simulink model "leader_follower"  (R2017b)
settings: Solver=FixedStepDiscrete  StartTime=0.0  StopTime=inf  FixedStep=0.1  RelTol=1e-3  EnableMultiTasking=on
undefined symbols (not defined in the file): Angular, Linear
libraries: robotlib x4, realtime_pacer_lib x1
settings Model: Creator=The MathWorks, Inc.  LastModifiedBy=bsb
settings DataIOCC: LimitDataPoints=on  SaveFormat=Array
settings OptimizationCC: DefaultUnderspecifiedDataType=single  LifeSpan=1  MaxStackSize=64
settings DebuggingCC: SolverPrmCheckMsg=warning  SFUnexpectedBacktrackingDiag=warning  SFNoUnconditionalDefaultTransitionDiag=warning  SFExecutionAtInitializationDiag=none
settings HardwareCC: ProdBitPerPointer=32  ProdBitPerSizeT=32  ProdBitPerPtrDiffT=32  ProdLargestAtomicFloat=None  ProdIntDivRoundTo=Undefined  ProdEndianess=Unspecified  ProdWordSize=32  ProdHWDeviceType=Generic->Unspecified (assume 32-bit Generic)  TargetHWDeviceType=Generic->Unspecified (assume 32-bit Generic)  UseEmbeddedCoderFeatures=off
settings ModelReferenceCC: PropagateSignalLabelsOutOfModel=off
settings RTWCC: SystemTargetFile=ert.tlc  HardwareBoard=Robot Operating System (ROS)  TLCOptions=-aInlineSetEventsForThisBaseRateFcn=TLC_FALSE -aSuppressMultiTaskScheduler=TLC_FALSE -aRateBasedStepFcn=0  TemplateMakefile=ert_default_tmf  Toolchain=Catkin  TargetLang=C++
settings CodeAppCC: StateflowObjectComments=on
settings ERTTargetCC: MultiwordLength=2048  ERTCustomFileBanners=off  MultiInstanceERTCode=on  CodeInterfacePackaging=C++ class  SupportContinuousTime=on  SupportNonInlinedSFcns=on  RemoveResetFunc=off  SupportVariableSizeSignals=on  ModelStepFunctionPrototypeControlCompliant=off  RootIOFormat=Structure reference  ConvertIfToSwitch=off  SuppressUnreachableDefaultCases=off
settings ConfigComp: CovMetricSettings=dw  CovHtmlReporting=on  CovSaveCumulativeToWorkspaceVar=on  CovSaveSingleToWorkspaceVar=on  CovExternalEMLEnable=off  CovSFcnEnable=off

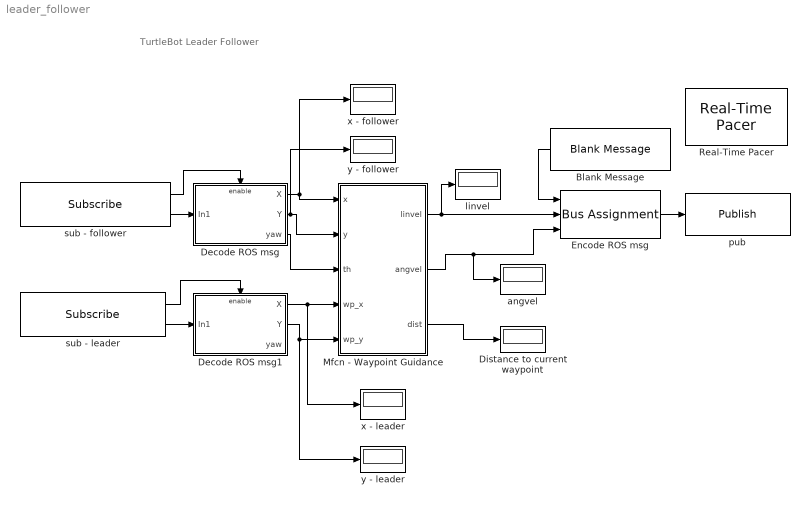
== system leader_follower ==
  note: TurtleBot Leader Follower
  Blank Message : robotlib/Blank Message  SourceLibraryInfo=This block requires Robotics System Toolbox  messageType=geometry_msgs/Twist  SampleTime=inf
      settings: SourceProductBaseCode=RO
  Decode ROS msg : Subsystem
  Decode ROS msg1 : Subsystem
  Distance to current waypoint : Display
  Encode ROS msg : BusAssignment  AssignedSignals=Linear.X,Angular.Z
  Mfcn - Waypoint Guidance : MATLAB Function  TreatAsAtomicUnit=on
  Real-Time Pacer : realtime_pacer_lib/Real-Time Pacer  simTimePerRealTime=1
  angvel : Display
  linvel : Display
  pub : robotlib/Publish  SourceLibraryInfo=This block requires Robotics System Toolbox  topicSource=Select from ROS network  topic=/tb3_1/cmd_vel  messageType=geometry_msgs/Twist  messageQueueLength=105
      settings: SourceProductBaseCode=RO
  "sub - follower " : robotlib/Subscribe  SourceLibraryInfo=This block requires Robotics System Toolbox  topicSource=Select from ROS network  topic=/tb3_1/amcl_pose  messageType=geometry_msgs/PoseWithCovarianceStamped  sampleTime=-1  messageQueueLength=51
      settings: SourceProductBaseCode=RO
  sub - leader : robotlib/Subscribe  SourceLibraryInfo=This block requires Robotics System Toolbox  topicSource=Select from ROS network  topic=/tb3_0/amcl_pose  messageType=geometry_msgs/PoseWithCovarianceStamped  sampleTime=-1  messageQueueLength=51
      settings: SourceProductBaseCode=RO
  x - follower : Display
  x - leader : Display
  y - follower : Display
  y - leader : Display
  wires:
  Encode ROS msg/1 -> pub/1
  "sub - follower "/1 -> Decode ROS msg/Enable
  "sub - follower "/2 -> Decode ROS msg/1(In1)
  Blank Message/1 -> Encode ROS msg/1
  Decode ROS msg/1(X) -> Mfcn - Waypoint Guidance/1(x), x - follower/1
  Decode ROS msg/2(Y) -> y - follower/1, Mfcn - Waypoint Guidance/2(y)
  Mfcn - Waypoint Guidance/3(dist) -> Distance to current waypoint/1
  Decode ROS msg1/1(X) -> x - leader/1, Mfcn - Waypoint Guidance/4(wp_x)
  Decode ROS msg/3(yaw) -> Mfcn - Waypoint Guidance/3(th)
  Mfcn - Waypoint Guidance/2(angvel) -> angvel/1, Encode ROS msg/3
  Mfcn - Waypoint Guidance/1(linvel) -> linvel/1, Encode ROS msg/2
  sub - leader/2 -> Decode ROS msg1/1(In1)
  Decode ROS msg1/2(Y) -> y - leader/1, Mfcn - Waypoint Guidance/5(wp_y)
  sub - leader/1 -> Decode ROS msg1/Enable

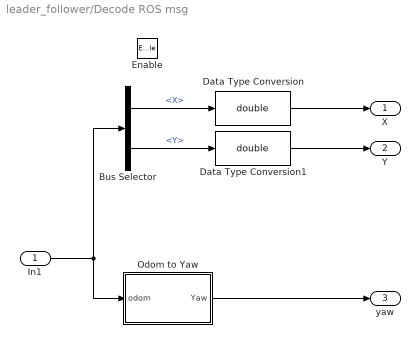
== system leader_follower/Decode ROS msg ==
  In1 : Inport
  Enable : EnablePort
  Bus Selector : BusSelector  DialogController=Simulink.DDGSource_BusSelector  OutputSignals=Pose.Pose.Position.X,Pose.Pose.Position.Y
  Data Type Conversion : DataTypeConversion  OutDataTypeStr=double
  Data Type Conversion1 : DataTypeConversion  OutDataTypeStr=double
  Odom to Yaw : Subsystem
  X : Outport
  Y : Outport  Port=2
  yaw : Outport  Port=3
  wires:
  In1/1 -> Odom to Yaw/1(odom), Bus Selector/1
  Bus Selector/2 -> Data Type Conversion1/1  "<Y>"
  Bus Selector/1 -> Data Type Conversion/1  "<X>"
  Data Type Conversion/1 -> X/1
  Data Type Conversion1/1 -> Y/1
  Odom to Yaw/1(Yaw) -> yaw/1

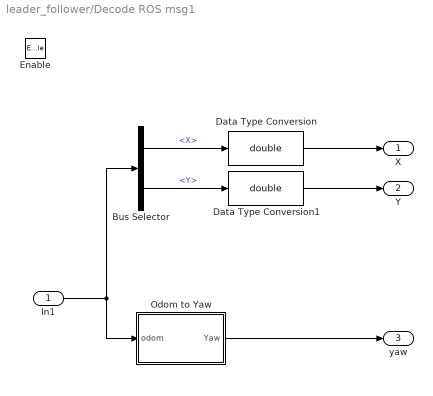
== system leader_follower/Decode ROS msg1 ==
  In1 : Inport
  Enable : EnablePort
  Bus Selector : BusSelector  DialogController=Simulink.DDGSource_BusSelector  OutputSignals=Pose.Pose.Position.X,Pose.Pose.Position.Y
  Data Type Conversion : DataTypeConversion  OutDataTypeStr=double
  Data Type Conversion1 : DataTypeConversion  OutDataTypeStr=double
  Odom to Yaw : Subsystem
  X : Outport
  Y : Outport  Port=2
  yaw : Outport  Port=3
  wires:
  In1/1 -> Odom to Yaw/1(odom), Bus Selector/1
  Bus Selector/2 -> Data Type Conversion1/1  "<Y>"
  Bus Selector/1 -> Data Type Conversion/1  "<X>"
  Data Type Conversion/1 -> X/1
  Data Type Conversion1/1 -> Y/1
  Odom to Yaw/1(Yaw) -> yaw/1

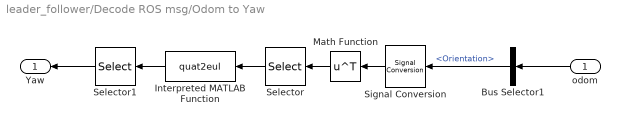
== system leader_follower/Decode ROS msg/Odom to Yaw ==
  odom : Inport
  Bus Selector1 : BusSelector  OutputSignals=Pose.Pose.Orientation
  Interpreted MATLAB Function : MATLABFcn  MATLABFcn=quat2eul  OutputDimensions=3
  Math Function : Math  Operator=transpose  SaturateOnIntegerOverflow=on
  Selector : Selector  InputPortWidth=4  IndexOptions=Index vector (dialog)  Indices=[4 1 2 3]  OutputSizes=1
  Selector1 : Selector  InputPortWidth=3  IndexOptions=Index vector (dialog)  Indices=1  OutputSizes=1
  Signal Conversion : SignalConversion  ConversionOutput=Virtual bus  OverrideOpt=off
  Yaw : Outport
  wires:
  odom/1 -> Bus Selector1/1
  Bus Selector1/1 -> Signal Conversion/1  "<Orientation>"
  Selector/1 -> Interpreted MATLAB Function/1
  Interpreted MATLAB Function/1 -> Selector1/1
  Selector1/1 -> Yaw/1
  Math Function/1 -> Selector/1
  Signal Conversion/1 -> Math Function/1

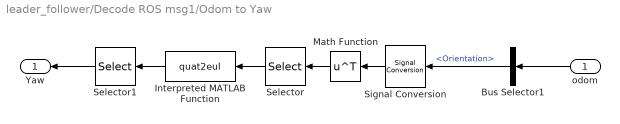
== system leader_follower/Decode ROS msg1/Odom to Yaw ==
  odom : Inport
  Bus Selector1 : BusSelector  OutputSignals=Pose.Pose.Orientation
  Interpreted MATLAB Function : MATLABFcn  MATLABFcn=quat2eul  OutputDimensions=3
  Math Function : Math  Operator=transpose  SaturateOnIntegerOverflow=on
  Selector : Selector  InputPortWidth=4  IndexOptions=Index vector (dialog)  Indices=[4 1 2 3]  OutputSizes=1
  Selector1 : Selector  InputPortWidth=3  IndexOptions=Index vector (dialog)  Indices=1  OutputSizes=1
  Signal Conversion : SignalConversion  ConversionOutput=Virtual bus  OverrideOpt=off
  Yaw : Outport
  wires:
  odom/1 -> Bus Selector1/1
  Bus Selector1/1 -> Signal Conversion/1  "<Orientation>"
  Selector/1 -> Interpreted MATLAB Function/1
  Interpreted MATLAB Function/1 -> Selector1/1
  Selector1/1 -> Yaw/1
  Math Function/1 -> Selector/1
  Signal Conversion/1 -> Math Function/1

== matlab function leader_follower/Mfcn - Waypoint Guidance ==
  data: linvel output; angvel output; x input; dist output; y input; th input; wp_x input; wp_y input
function [linvel,angvel,dist] = wpt_fcn(x,y,th,wp_x,wp_y)
% Function to implement waypoint guidance
% Inputs:
%  - x: Current X position
%  - y: Current Y position
%  - th: Current theta position
%  - wp_x: Current waypoint goals, X
%  - wp_y: Current waypoint goals, X
% Outputs:
%  - dist: Distance from current position to current waypoint goal
%  - angvel: Desired angular velocity [rad/s, clockwise]
%  - linvel: Desired linear velocity


% Distance from waypoint to current location
dist = sqrt((x-wp_x)^2+(y-wp_y)^2);

% Angle from current location to waypoint
course = atan2(wp_y-y,wp_x-x);

% Difference (error) between current turtle angle and desired angle
dhdg = course-th;

% Unwrap angle
while dhdg < -pi
    dhdg = dhdg + 2*pi;
end
while dhdg > pi
    dhdg = dhdg - 2*pi;
end

% Proportional Control
% Gains
Kpvel = 1.5;  % Proportional gain for velocity
Kphdg = 1.0;  % Proportional gain for heading

% Specify commands to turtle
angvel=Kphdg*dhdg;
linvel = Kpvel*dist;

% Limit the maximum linear velocity
maxlv = 1.5;
if abs(linvel) > maxlv
    linvel = sign(linvel)*maxlv;
end

% Turn only if large heading error
if abs(dhdg) > 45.0*pi/180;
    linvel = 0.0;  %0.1*linvel;
end

end
